simulink library "TimestampChecker"  (R2016b)
settings: Solver=VariableStepAuto  StartTime=0.0  StopTime=10.0  RelTol=1e-3
settings Model: Creator=Nathan  LastModifiedBy=march

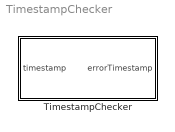
== system TimestampChecker ==
  TimestampChecker : Subsystem

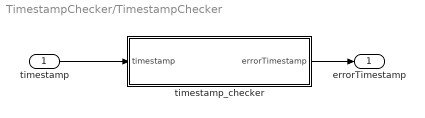
== system TimestampChecker/TimestampChecker ==
  timestamp : Inport
  timestamp_checker : MATLAB Function  TreatAsAtomicUnit=on
  errorTimestamp : Outport
  wires:
  timestamp_checker/1(errorTimestamp) -> errorTimestamp/1
  timestamp/1 -> timestamp_checker/1(timestamp)

== matlab function TimestampChecker/timestamp_checker ==
  data: timestamp input; errorTimestamp output
function errorTimestamp = timestamp_checker(timestamp)
maxNonResponsive = 0.3; %[seconds]
sampleTime = 0.002; %[seconds]

persistent lastTimestamp;
persistent nonResponsive;

%Initialize error and lastTimestamp if models starts
if(isempty(lastTimestamp))
    lastTimestamp = 0;
    nonResponsive = 0;
end

if((timestamp == lastTimestamp))
    nonResponsive = nonResponsive + 1;
    errorTimestamp = 0;
    %Checks if the timestamp is the same as lastTimestamp, which means
    %that the SOMANET has not update and thus is not responding
    
elseif(nonResponsive*sampleTime >= maxNonResponsive)
    errorTimestamp = 1;
    %Checks if the SOMANET has not responded for longer than the maximum
    %allowed non responsive time.
    
else
    lastTimestamp = timestamp;
    nonResponsive = 0;
    errorTimestamp = 0;
end


end
